simulink model "TCLab_PID_FF"  (Simulink 10.3)
settings: Solver=ode45  StartTime=0.0  StopTime=2000  FixedStep=0.1  RelTol=1e-3  EnableMultiTasking=on
PreLoadFcn:
  | variables
values from neighbouring files (symbols this model uses):
  Ts = 1    [variables.m]
libraries: Process x1
settings Model: Creator=auto2  LastModifiedBy=thibaut  MultithreadedSim=on  ExtModeTrigMode=oneshot  ExtModeArmWhenConnect=off
settings DataIOCC: SaveOutput=off  SaveTime=off  SignalLoggingName=sigsOut
settings OptimizationCC: BooleanDataType=off  InitFltsAndDblsToZero=on
settings DebuggingCC: SaveWithParameterizedLinksMsg=none  SignalResolutionControl=TryResolveAllWithWarning  MultiTaskDSMMsg=warning  MultiTaskCondExecSysMsg=none  PregeneratedLibrarySubsystemCodeDiagnostic=none
settings HardwareCC: TargetUnknown=on
settings ConfigComp: CovSFcnEnable=off

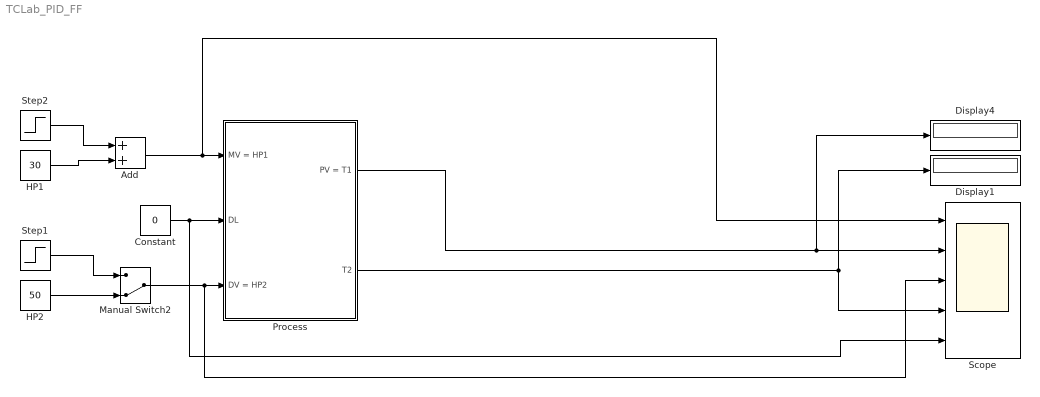
== system TCLab_PID_FF ==
  Add : Sum
  Constant : Constant  Value=0
  Display1 : Display
  Display4 : Display
  HP1 : Constant  Value=30  SampleTime=Ts
  HP2 : Constant  Value=50  SampleTime=Ts
  Manual Switch2 : ManualSwitch  CurrentSetting=0
  Process : Subsystem  BlockChoice=TCLab_model
      settings: AttributesFormatString=%<BlockChoice>  TemplateBlock=Process/Process  MemberBlocks=TCLab,TCLab_model
  Scope : Scope  NumInputPorts=5
  Step1 : Step  Time=300  Before=50  After=60  SampleTime=Ts
  Step2 : Step  Time=800  After=40  SampleTime=Ts
  wires:
  Manual Switch2/1 -> Process/3(DV = HP2), Scope/3
  Add/1 -> Scope/1, Process/1(MV = HP1)
  Process/1(PV = T1) -> Display4/1, Scope/2
  Process/2(T2) -> Scope/4, Display1/1
  Step1/1 -> Manual Switch2/1
  HP2/1 -> Manual Switch2/2
  Constant/1 -> Scope/5, Process/2(DL)
  Step2/1 -> Add/1
  HP1/1 -> Add/2

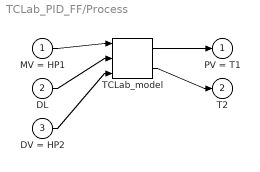
== system TCLab_PID_FF/Process ==
  MV = HP1 : Inport
  DL : Inport  Port=2
  DV = HP2 : Inport  Port=3
  TCLab_model : Process/TCLab_model  SystemSampleTime=-1  VariantActivationTime=update diagram  Latency=0  AutoFrameSizeCalculation=off
  PV = T1 : Outport  VectorParamsAs1DForOutWhenUnconnected=off
  T2 : Outport  Port=2  VectorParamsAs1DForOutWhenUnconnected=off
  wires:
  MV = HP1/1 -> TCLab_model/1
  DL/1 -> TCLab_model/2
  DV = HP2/1 -> TCLab_model/3
  TCLab_model/1 -> PV = T1/1
  TCLab_model/2 -> T2/1
